simulink model "s_VI_exact_control_pid_OL_14bb"  (Simulink 8.4)
settings: Solver=ode45  SolverMode=SingleTasking  StartTime=0.0  StopTime=10.0  RelTol=1e-3
values from neighbouring files (symbols this model uses):
  Kd = 80    [m_IV_run_pid_contr.m]
  Ki = 200    [m_IV_run_pid_contr.m]
  Kp = 500    [m_IV_run_pid_contr.m]
settings Model: Creator=a_bad  LastModifiedBy=a_bad  CovMetricSettings=dwe  CovHtmlReporting=off  covSaveCumulativeToWorkspaceVar=off  CovSaveSingleToWorkspaceVar=off  CovExternalEMLEnable=on  CovSFcnEnable=on
settings DataIOCC: LimitDataPoints=off  SaveFormat=StructureWithTime  SignalLoggingSaveFormat=Dataset
settings OptimizationCC: ExpressionDepthLimit=128
settings DebuggingCC: AlgebraicLoopMsg=none  UnderspecifiedInitializationDetection=Simplified  MergeDetectMultiDrivingBlocksExec=error  SolverPrmCheckMsg=none  FcnCallInpInsideContextMsg=EnableAllAsError  FrameProcessingCompatibilityMsg=error  StateNameClashWarn=none  SFUnexpectedBacktrackingDiag=error  SFNoUnconditionalDefaultTransitionDiag=error
settings HardwareCC: ProdBitPerPointer=64  ProdLargestAtomicFloat=Float  ProdIntDivRoundTo=Zero  ProdEndianess=LittleEndian  ProdHWDeviceType=Specified
settings ModelReferenceCC: PropagateSignalLabelsOutOfModel=on
settings GRTTargetCC: TargetLangStandard=C99 (ISO)  GeneratePreprocessorConditionals=Use local settings  CombineOutputUpdateFcns=on  GRTInterface=off

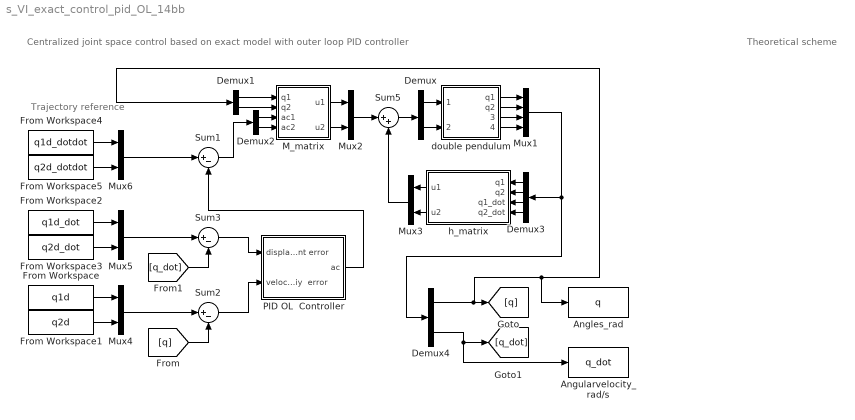
== system s_VI_exact_control_pid_OL_14bb ==
  note: Theoretical scheme
  note: Trajectory
      | reference
  note: Centralized joint space control based on exact model with outer loop PID controller
  Angles_rad : ToWorkspace  VariableName=q  SaveFormat=Timeseries  SampleTime=-1
  Angularvelocity_rad/s : ToWorkspace  VariableName=q_dot  SaveFormat=Timeseries  SampleTime=-1
  Demux{,1..2,4} (4 alike) : Demux  Outputs=2
  Demux3 : Demux
  From Workspace : FromWorkspace  VariableName=q1d  SampleTime=0
  From Workspace1 : FromWorkspace  VariableName=q2d  SampleTime=0
  From Workspace2 : FromWorkspace  VariableName=q1d_dot  SampleTime=0
  From Workspace3 : FromWorkspace  VariableName=q2d_dot  SampleTime=0
  From Workspace4 : FromWorkspace  VariableName=q1d_dotdot  SampleTime=0
  From Workspace5 : FromWorkspace  VariableName=q2d_dotdot  SampleTime=0
  "M_matrix " : MATLAB Function  TreatAsAtomicUnit=on
      settings: PermitHierarchicalResolution=ParametersOnly
  Mux1 : Mux
  Mux{2..6} (5 alike) : Mux  Inputs=2
  PID OL  Controller : Subsystem
  Sum1 : Sum  Inputs=|+-
  Sum2 : Sum  Inputs=|+-
  Sum3 : Sum  Inputs=|+-
  Sum5 : Sum  Inputs=|++
  "double pendulum " : Subsystem
      mask Display: image('294px-Double-Pendulum.svg.png');
  "h_matrix " : MATLAB Function  TreatAsAtomicUnit=on
      settings: PermitHierarchicalResolution=ParametersOnly
  wires:
  "double pendulum "/1(q1) -> Mux1/1
  Demux/1 -> "double pendulum "/1(Tau1)
  Demux/2 -> "double pendulum "/2("Tau2 ")
  "M_matrix "/2(u2) -> Mux2/2
  "M_matrix "/1(u1) -> Mux2/1
  "h_matrix "/1(u1) -> Mux3/1
  "h_matrix "/2(u2) -> Mux3/2
  Demux3/1 -> "h_matrix "/1(q1)
  Demux3/2 -> "h_matrix "/2(q2)
  Demux3/3 -> "h_matrix "/3(q1_dot)
  Demux3/4 -> "h_matrix "/4(q2_dot)
  "double pendulum "/4(q2_dot) -> Mux1/4
  "double pendulum "/2("q2  ") -> Mux1/2
  "double pendulum "/3("q1_dot ") -> Mux1/3
  Mux1/1 -> Demux4/1, Demux3/1
  Demux1/1 -> "M_matrix "/1(q1)
  Demux1/2 -> "M_matrix "/2(q2)
  Demux4/2 -> Angularvelocity_rad/s/1, [q_dot]
  [q] -> Sum2/2
  [q_dot] -> Sum3/2
  Demux4/1 -> Demux1/1, Angles_rad/1, [q]
  From Workspace/1 -> Mux4/1
  From Workspace1/1 -> Mux4/2
  Mux4/1 -> Sum2/1
  From Workspace2/1 -> Mux5/1
  From Workspace3/1 -> Mux5/2
  Mux5/1 -> Sum3/1
  From Workspace5/1 -> Mux6/2
  From Workspace4/1 -> Mux6/1
  Demux2/2 -> "M_matrix "/4(ac2)
  Sum1/1 -> Demux2/1
  Demux2/1 -> "M_matrix "/3(ac1)
  Mux6/1 -> Sum1/1
  Mux2/1 -> Sum5/1
  Mux3/1 -> Sum5/2
  Sum5/1 -> Demux/1
  Sum3/1 -> PID OL  Controller/1(displacement error)
  Sum2/1 -> PID OL  Controller/2(veloctiy  error)
  PID OL  Controller/1(ac) -> Sum1/2

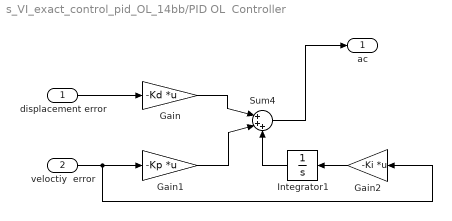
== system s_VI_exact_control_pid_OL_14bb/PID OL  Controller ==
  displacement error : Inport
  veloctiy  error : Inport  Port=2
  Gain : Gain  Gain=-Kd  Multiplication=Matrix(K*u)
  Gain1 : Gain  Gain=-Kp  Multiplication=Matrix(K*u)
  Gain2 : Gain  Gain=-Ki  Multiplication=Matrix(K*u)
  Integrator1 : Integrator
  Sum4 : Sum  Inputs=|+++
  ac : Outport
  wires:
  Sum4/1 -> ac/1
  Gain1/1 -> Sum4/2
  displacement error/1 -> Gain/1
  Gain/1 -> Sum4/1
  Gain2/1 -> Integrator1/1
  veloctiy  error/1 -> Gain2/1, Gain1/1
  Integrator1/1 -> Sum4/3

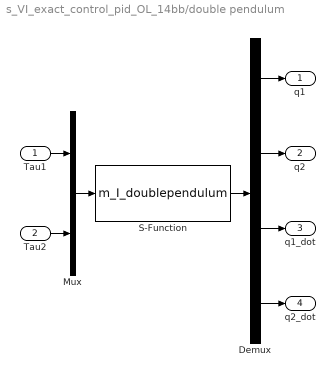
== system s_VI_exact_control_pid_OL_14bb/double pendulum  ==
  Tau1 : Inport
  "Tau2 " : Inport  Port=2
  Demux : Demux
  Mux : Mux  Inputs=2
  S-Function : S-Function  FunctionName=m_I_doublependulum  Parameters=0 0 0 0  SFunctionDeploymentMode=off  EnableBusSupport=off
  q1 : Outport
  "q2  " : Outport  Port=2
  "q1_dot " : Outport  Port=3
  q2_dot : Outport  Port=4
  wires:
  Mux/1 -> S-Function/1
  S-Function/1 -> Demux/1
  Tau1/1 -> Mux/1
  "Tau2 "/1 -> Mux/2
  Demux/4 -> q2_dot/1
  Demux/3 -> "q1_dot "/1
  Demux/2 -> "q2  "/1
  Demux/1 -> q1/1

== matlab function M_matrix  ==
  data: q1 input double; q2 input double; ac1 input double; u1 output double; ac2 input double; u2 output double
function [u1,u2] = fcn(q1,q2,ac1,ac2)
Grav=10;     %%Gravity acceleration constant
M=1;       
L1=1;
L2=1;
Gz=1;
beta=20;
Ts=0.01;    %%sampling time
G1=M*(L1^2+L2^2)+Gz;
G2=M*L2^2+Gz;
H11=G1+2*M*L1*L2*cos(q2);   H12=G2+  M*L1*L2*cos(q2);
H21=G2+  M*L1*L2*cos(q2);   H22=G2;

u1= H11*ac1+H12*ac2;
u2= H21*ac1+H22*ac2;

== matlab function h_matrix  ==
  data: q1 input double; u1 output double; q2 input double; q1_dot input double; q2_dot input double; u2 output double
function [u1,u2] = fcn(q1,q2,q1_dot,q2_dot)
Grav=10;     %%Gravity acceleration constant
M=1;       
L1=1;
L2=1;
Gz=1;
beta=20;
G1=M*(L1^2+L2^2)+Gz;
G2=M*L2^2+Gz;
C11=-2*M*L1*L2*sin(q2)*q2_dot;  C12=-M*L1*L2*cos(q2)*q2_dot;
C21=M*L1*L2*sin(q2)*q1_dot;     C22=0;
g1=M*Grav*(L1*cos(q1)+L2*cos(q1+q2));    g2=M*Grav*L2*cos(q1+q2);
u1=[C11 C12]*[q1_dot;q2_dot]+g1+[beta 0]*[q1_dot;q2_dot];
u2=[C21 C22]*[q1_dot;q2_dot]+g2+[0 beta]*[q1_dot;q2_dot];
